simulink model "ipmsm_current_control_CV_FF"  (R2023a)
settings: Solver=FixedStepDiscrete  StartTime=0.0  StopTime=0.8  FixedStep=Ts  RelTol=1e-3  EnableMultiTasking=on
PreLoadFcn:
  | ee_ipmsm_velocity_control_data;
StopFcn:
  | ee_addSimlogTimeStamp(bdroot)
values from neighbouring files (symbols this model uses):
  ActCV = 1    [ipmsm_current_control_data.m]
  down1 = den(1)    [ipmsm_current_control_data.m]
  down2 = den(2)    [ipmsm_current_control_data.m]
  Ki_id = 0.6*Ld/(5*sigma*sigma)    (= 3750)    [ipmsm_current_control_data.m]
  Ki_iq = 0.6*Lq/(5*sigma*sigma)    (= 3750)    [ipmsm_current_control_data.m]
  Kp_id = 0.6*Ld/sigma    (= 1.5)    [ipmsm_current_control_data.m]
  Kp_iq = 0.6*Lq/sigma    (= 1.5)    [ipmsm_current_control_data.m]
  Ld = 0.2e-3    (= 0.0002)    [ipmsm_current_control_data.m]
  Lq = 0.2e-3    (= 0.0002)    [ipmsm_current_control_data.m]
  p = 4    [ipmsm_current_control_data.m]
  Pmax = 1.2*445.3845    (= 534.4614)    [ipmsm_current_control_data.m]
  psim = 0.0064    [ipmsm_current_control_data.m]
  Tmax = 1.2*0.8223    (= 0.98676)    [ipmsm_current_control_data.m]
  Ts = 1e-6    (= 1e-06)    [ipmsm_current_control_data.m]
  Tsi = 5e-5    (= 5e-05)    [ipmsm_current_control_data.m]
  up = num(2)    [ipmsm_current_control_data.m]
  Vnom = 24    [ipmsm_current_control_data.m]
undefined symbols (not defined in the file or in its folder): ee_sli_rtmsupport, gcbh, ID_MAP, IQ_MAP, RPM_VECT, TQ_VECT, VDC_VECT
libraries: nesl_utility x13, fl_lib x10, simulink x10, ee_lib x5, spsMeanLib x4, slpidlib x2, eeDiscretePi x2, eeTransforms x2, eeVelocityController x1, eePwmGeneratorTwoLevel x1, SignalEditorBlockLib x1
(part 2 of 2)

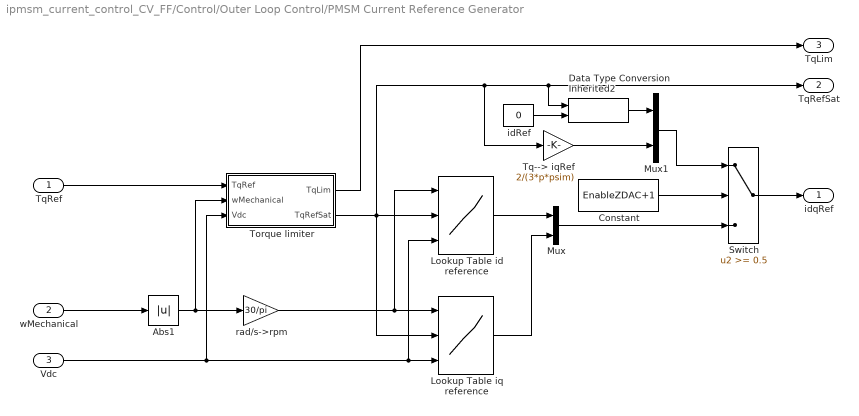
== system ipmsm_current_control_CV_FF/Control/Outer Loop Control/PMSM Current Reference Generator ==
  TqRef : Inport  SampleTime=Ts
  wMechanical : Inport  Port=2  SampleTime=Ts
  Vdc : Inport  Port=3  SampleTime=Ts
  Abs1 : Abs  SaturateOnIntegerOverflow=off
  Constant : Constant  Value=EnableZDAC+1  SampleTime=Ts
  Data Type Conversion Inherited2 : simulink/Signal Attributes/Data Type Conversion Inherited  ConvertRealWorld=Real World Value  DoSatur=off
  Lookup Table id reference : Lookup_n-D  NumberOfTableDimensions=3  BreakpointsForDimension1=rpmVec  BreakpointsForDimension2=TqVec  BreakpointsForDimension3=VdcVec  Table=idMatrix
      settings: InputPortMap=u0,u1,u2
  Lookup Table iq reference : Lookup_n-D  NumberOfTableDimensions=3  BreakpointsForDimension1=rpmVec  BreakpointsForDimension2=TqVec  BreakpointsForDimension3=VdcVec  Table=iqMatrix
      settings: InputPortMap=u0,u1,u2
  Mux : Mux  Inputs=2
  Mux1 : Mux  Inputs=2
  Switch : Switch  Threshold=0.5  SaturateOnIntegerOverflow=off  InputSameDT=off
  Torque limiter : Subsystem
  Tq--> iqRef : Gain  Gain=2/(3*p*psim)
  idRef : Constant  Value=0  SampleTime=Ts
  rad/s->rpm : Gain  Gain=30/pi
  idqRef : Outport  VectorParamsAs1DForOutWhenUnconnected=off
  TqRefSat : Outport  Port=2  VectorParamsAs1DForOutWhenUnconnected=off
  TqLim : Outport  Port=3  VectorParamsAs1DForOutWhenUnconnected=off
  wires:
  idRef/1 -> Data Type Conversion Inherited2/2
  Lookup Table id reference/1 -> Mux/1
  Lookup Table iq reference/1 -> Mux/2
  Torque limiter/2(TqRefSat) -> Lookup Table iq reference/2, Tq--> iqRef/1, TqRefSat/1, Data Type Conversion Inherited2/1, Lookup Table id reference/2
  Torque limiter/1(TqLim) -> TqLim/1
  rad/s->rpm/1 -> Lookup Table id reference/1, Lookup Table iq reference/1
  Abs1/1 -> Torque limiter/2(wMechanical), rad/s->rpm/1
  Mux1/1 -> Switch/1
  Mux/1 -> Switch/3
  Switch/1 -> idqRef/1
  Data Type Conversion Inherited2/1 -> Mux1/1
  Tq--> iqRef/1 -> Mux1/2
  TqRef/1 -> Torque limiter/1(TqRef)
  wMechanical/1 -> Abs1/1
  Vdc/1 -> Lookup Table id reference/3, Lookup Table iq reference/3, Torque limiter/3(Vdc)
  Constant/1 -> Switch/2

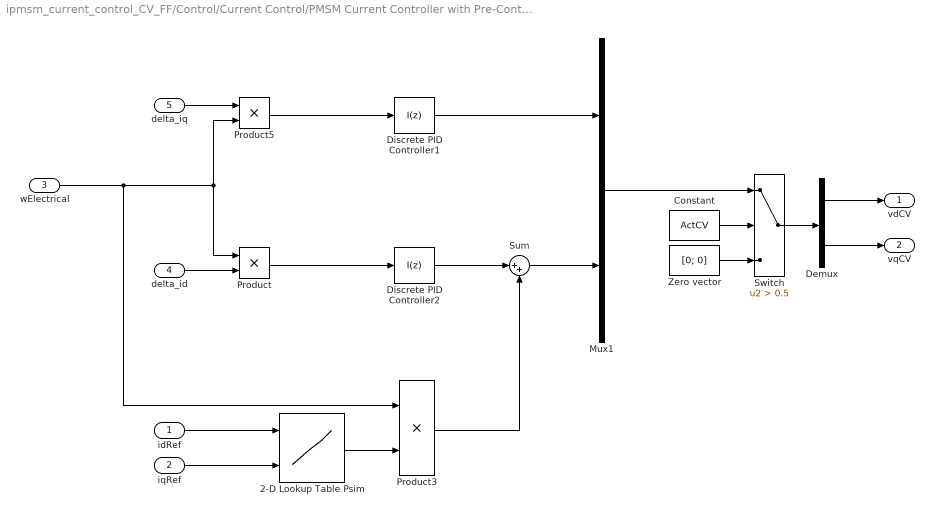
== system ipmsm_current_control_CV_FF/Control/Current Control/PMSM Current Controller with Pre-Control and CV Decoupling/Complex Vector Decoupling ==
  idRef : Inport
  iqRef : Inport  Port=2
  wElectrical : Inport  Port=3
  delta_id : Inport  Port=4
  delta_iq : Inport  Port=5
  2-D Lookup Table Psim : Lookup_n-D  BreakpointsForDimension1=idVect  BreakpointsForDimension2=iqVect  Table=psimMatrix  ExtrapMethod=Clip  InternalRulePriority=Speed  RndMeth=Simplest
      settings: InputPortMap=u0,u1
  Constant : Constant  Value=ActCV  SampleTime=Ts
  Demux : Demux  Outputs=2
  Discrete PID Controller1 : slpidlib/PID Controller  Controller=I  Form=Parallel  TimeDomain=Discrete-time  UseExternalTs=off  SampleTime=Ts  IntegratorMethod=Forward Euler  FilterMethod=Forward Euler  ControllerParametersSource=internal  P=0  I=Kp_iq  UseKiTs=off  D=0  N=100  UseFilter=on  TunerSelectOption=Transfer Function Based (PID Tuner App)  InitialConditionSource=internal  InitialConditionForIntegrator=0  InitialConditionForFilter=0  DifferentiatorICPrevScaledInput=0  ExternalReset=none  TrackingMode=off  Kt=1  LimitOutput=on  SatLimitsSource=internal  UpperSaturationLimit=146.25  LowerSaturationLimit=-146.25  LinearizeAsGain=off  AntiWindupMode=none  Kb=1  LimitIntegrator=off  UpperIntegratorSaturationLimit=inf  LowerIntegratorSaturationLimit=-inf  POutMin=[]  POutMax=[]  IOutMin=[]  IOutMax=[]  DOutMin=[]  DOutMax=[]  NOutMin=[]  NOutMax=[]  SumOutMin=[]  SumOutMax=[]  SaturationOutMin=[]  SaturationOutMax=[]  PParamMin=[]  PParamMax=[]  IParamMin=[]  IParamMax=[]  DParamMin=[]  DParamMax=[]  NParamMin=[]  NParamMax=[]  KbParamMin=[]  KbParamMax=[]  KtParamMin=[]  KtParamMax=[]  KbOutMin=[]  KbOutMax=[]  KtOutMin=[]  KtOutMax=[]  IntegratorOutMin=[]  IntegratorOutMax=[]  FilterOutMin=[]  FilterOutMax=[]  SumI1OutMin=[]  SumI1OutMax=[]  SumI2OutMin=[]  SumI2OutMax=[]  SumI3OutMin=[]  SumI3OutMax=[]  SumI4OutMin=[]  SumI4OutMax=[]  SumDOutMin=[]  SumDOutMax=[]  DifferentiatorOutMin=[]  DifferentiatorOutMax=[]  FilterDiffOutCoefMin=[]  FilterDiffOutCoefMax=[]  ReciprocalOutMin=[]  ReciprocalOutMax=[]  SumDenOutMin=[]  SumDenOutMax=[]  SumNumOutMin=[]  SumNumOutMax=[]  DivideOutMin=[]  DivideOutMax=[]  UdiffTsProdOutMin=[]  UdiffTsProdOutMax=[]  NTsProdOutMin=[]  NTsProdOutMax=[]  UintegralTsProdOutMin=[]  UintegralTsProdOutMax=[]  UngainTsProdOutMin=[]  UngainTsProdOutMax=[]  ClampingZeroOutDataTypeStr=Inherit: Inherit via back propagation  ClampingZeroOutMin=[]  ClampingZeroOutMax=[]  FilterDenConstantOutDataTypeStr=Inherit: Inherit via back propagation  FilterDenConstantOutMin=[]  FilterDenConstantOutMax=[]  PCopyOutDataTypeStr=Inherit: Inherit via back propagation  PCopyOutMin=[]  PCopyOutMax=[]  NCopyOutDataTypeStr=Inherit: Inherit via back propagation  NCopyOutMin=[]  NCopyOutMax=[]  IntegratorContinuousStateAttributes=''  IntegratorStateMustResolveToSignalObject=off  IntegratorRTWStateStorageClass=Auto  FilterContinuousStateAttributes=''  FilterStateMustResolveToSignalObject=off  FilterRTWStateStorageClass=Auto  ParallelPVariant=Disabled  IdealPVariant=Disabled  IVariant=InternalParameters  DVariant=Disabled  IntegratorVariant=Discrete  SatVariant=Enabled  AWVariant=Passthrough  PCopyVariant=Disabled  TRVariant=Disabled  FdbkBlocksVariant=Forward  IdealPFdbkVariant=Disabled  SatFdbkVariant=Disabled  DerivativeFilterVariant=Disabled  NVariant=Disabled  NCopyVariant=Disabled_SignalSpec  FilterICVariant=Disabled  IntegratorICVariant=InternalICs  ExternalResetVariant=Disabled  TRSumVariant=Passthrough  SumFdbkVariant=Disabled  SumVariant=Passthrough_I  TsampFilterVariant=InternalTs  TsampNgainVariant=Passthrough  TsampIntegralVariant=Disabled_SignalSpec  ExternalSaturationOutDataTypeStr=Inherit: Same as second input
  Discrete PID Controller2 : slpidlib/PID Controller  Controller=I  Form=Parallel  TimeDomain=Discrete-time  UseExternalTs=off  SampleTime=Ts  IntegratorMethod=Forward Euler  FilterMethod=Forward Euler  ControllerParametersSource=internal  P=0  I=Kp_id  UseKiTs=off  D=0  N=100  UseFilter=on  TunerSelectOption=Transfer Function Based (PID Tuner App)  InitialConditionSource=internal  InitialConditionForIntegrator=0  InitialConditionForFilter=0  DifferentiatorICPrevScaledInput=0  ExternalReset=none  TrackingMode=off  Kt=1  LimitOutput=on  SatLimitsSource=internal  UpperSaturationLimit=146.25  LowerSaturationLimit=-146.25  LinearizeAsGain=off  AntiWindupMode=none  Kb=1  LimitIntegrator=off  UpperIntegratorSaturationLimit=inf  LowerIntegratorSaturationLimit=-inf  POutMin=[]  POutMax=[]  IOutMin=[]  IOutMax=[]  DOutMin=[]  DOutMax=[]  NOutMin=[]  NOutMax=[]  SumOutMin=[]  SumOutMax=[]  SaturationOutMin=[]  SaturationOutMax=[]  PParamMin=[]  PParamMax=[]  IParamMin=[]  IParamMax=[]  DParamMin=[]  DParamMax=[]  NParamMin=[]  NParamMax=[]  KbParamMin=[]  KbParamMax=[]  KtParamMin=[]  KtParamMax=[]  KbOutMin=[]  KbOutMax=[]  KtOutMin=[]  KtOutMax=[]  IntegratorOutMin=[]  IntegratorOutMax=[]  FilterOutMin=[]  FilterOutMax=[]  SumI1OutMin=[]  SumI1OutMax=[]  SumI2OutMin=[]  SumI2OutMax=[]  SumI3OutMin=[]  SumI3OutMax=[]  SumI4OutMin=[]  SumI4OutMax=[]  SumDOutMin=[]  SumDOutMax=[]  DifferentiatorOutMin=[]  DifferentiatorOutMax=[]  FilterDiffOutCoefMin=[]  FilterDiffOutCoefMax=[]  ReciprocalOutMin=[]  ReciprocalOutMax=[]  SumDenOutMin=[]  SumDenOutMax=[]  SumNumOutMin=[]  SumNumOutMax=[]  DivideOutMin=[]  DivideOutMax=[]  UdiffTsProdOutMin=[]  UdiffTsProdOutMax=[]  NTsProdOutMin=[]  NTsProdOutMax=[]  UintegralTsProdOutMin=[]  UintegralTsProdOutMax=[]  UngainTsProdOutMin=[]  UngainTsProdOutMax=[]  ClampingZeroOutDataTypeStr=Inherit: Inherit via back propagation  ClampingZeroOutMin=[]  ClampingZeroOutMax=[]  FilterDenConstantOutDataTypeStr=Inherit: Inherit via back propagation  FilterDenConstantOutMin=[]  FilterDenConstantOutMax=[]  PCopyOutDataTypeStr=Inherit: Inherit via back propagation  PCopyOutMin=[]  PCopyOutMax=[]  NCopyOutDataTypeStr=Inherit: Inherit via back propagation  NCopyOutMin=[]  NCopyOutMax=[]  IntegratorContinuousStateAttributes=''  IntegratorStateMustResolveToSignalObject=off  IntegratorRTWStateStorageClass=Auto  FilterContinuousStateAttributes=''  FilterStateMustResolveToSignalObject=off  FilterRTWStateStorageClass=Auto  ParallelPVariant=Disabled  IdealPVariant=Disabled  IVariant=InternalParameters  DVariant=Disabled  IntegratorVariant=Discrete  SatVariant=Enabled  AWVariant=Passthrough  PCopyVariant=Disabled  TRVariant=Disabled  FdbkBlocksVariant=Forward  IdealPFdbkVariant=Disabled  SatFdbkVariant=Disabled  DerivativeFilterVariant=Disabled  NVariant=Disabled  NCopyVariant=Disabled_SignalSpec  FilterICVariant=Disabled  IntegratorICVariant=InternalICs  ExternalResetVariant=Disabled  TRSumVariant=Passthrough  SumFdbkVariant=Disabled  SumVariant=Passthrough_I  TsampFilterVariant=InternalTs  TsampNgainVariant=Passthrough  TsampIntegralVariant=Disabled_SignalSpec  ExternalSaturationOutDataTypeStr=Inherit: Same as second input
  Mux1 : Mux  Inputs=2
  Product : Product
  Product3 : Product
  Product5 : Product
  Sum : Sum  Inputs=|++
  Switch : Switch  Criteria=u2 > Threshold  Threshold=0.5  SaturateOnIntegerOverflow=off  InputSameDT=off  OutDataTypeStr=Inherit: Same as first input
  Zero vector : Constant  Value=[0; 0]  SampleTime=Ts
  vdCV : Outport  VectorParamsAs1DForOutWhenUnconnected=off
  vqCV : Outport  Port=2  VectorParamsAs1DForOutWhenUnconnected=off
  wires:
  Switch/1 -> Demux/1
  Demux/2 -> vqCV/1
  Constant/1 -> Switch/2
  Mux1/1 -> Switch/1
  Demux/1 -> vdCV/1
  Zero vector/1 -> Switch/3
  Product/1 -> Discrete PID Controller2/1
  Product5/1 -> Discrete PID Controller1/1
  Discrete PID Controller2/1 -> Sum/1
  idRef/1 -> 2-D Lookup Table Psim/1
  iqRef/1 -> 2-D Lookup Table Psim/2
  delta_iq/1 -> Product5/1
  delta_id/1 -> Product/2
  wElectrical/1 -> Product3/1, Product/1, Product5/2
  2-D Lookup Table Psim/1 -> Product3/2
  Product3/1 -> Sum/2
  Sum/1 -> Mux1/2
  Discrete PID Controller1/1 -> Mux1/1

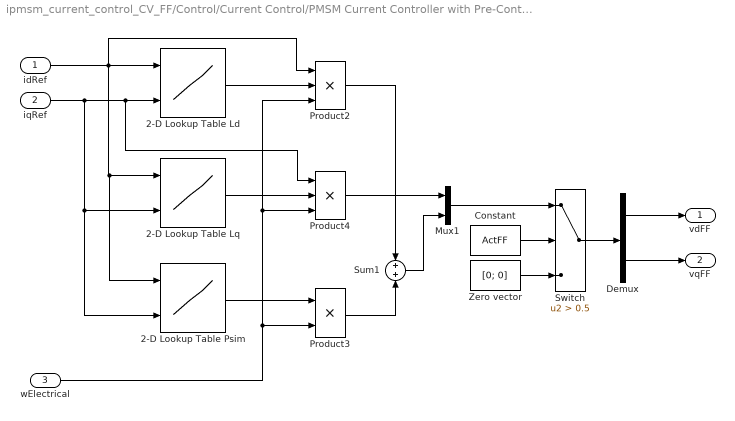
== system ipmsm_current_control_CV_FF/Control/Current Control/PMSM Current Controller with Pre-Control and CV Decoupling/Feedforward pre-control ==
  idRef : Inport
  iqRef : Inport  Port=2
  wElectrical : Inport  Port=3
  2-D Lookup Table Ld : Lookup_n-D  BreakpointsForDimension1=idVect  BreakpointsForDimension2=iqVect  Table=LdMatrix  ExtrapMethod=Clip  UseLastTableValue=on  InternalRulePriority=Speed  RndMeth=Simplest
      settings: InputPortMap=u0,u1
  2-D Lookup Table Lq : Lookup_n-D  BreakpointsForDimension1=idVect  BreakpointsForDimension2=iqVect  Table=LqMatrix  ExtrapMethod=Clip  InternalRulePriority=Speed  RndMeth=Simplest
      settings: InputPortMap=u0,u1
  2-D Lookup Table Psim : Lookup_n-D  BreakpointsForDimension1=idVect  BreakpointsForDimension2=iqVect  Table=psimMatrix  ExtrapMethod=Clip  InternalRulePriority=Speed  RndMeth=Simplest
      settings: InputPortMap=u0,u1
  Constant : Constant  Value=ActFF  SampleTime=Ts
  Demux : Demux  Outputs=2
  Mux1 : Mux  Inputs=2
  Product2 : Product  Inputs=3
  Product3 : Product
  Product4 : Product  Inputs=3
  Sum1 : Sum
  Switch : Switch  Criteria=u2 > Threshold  Threshold=0.5  SaturateOnIntegerOverflow=off  InputSameDT=off  OutDataTypeStr=Inherit: Same as first input
  Zero vector : Constant  Value=[0; 0]  SampleTime=Ts
  vdFF : Outport  VectorParamsAs1DForOutWhenUnconnected=off
  vqFF : Outport  Port=2  VectorParamsAs1DForOutWhenUnconnected=off
  wires:
  Product2/1 -> Sum1/1
  wElectrical/1 -> Product2/3, Product4/3, Product3/2
  Mux1/1 -> Switch/1
  Product4/1 -> Mux1/1
  idRef/1 -> 2-D Lookup Table Ld/1, 2-D Lookup Table Lq/1, 2-D Lookup Table Psim/1, Product2/1
  iqRef/1 -> 2-D Lookup Table Psim/2, 2-D Lookup Table Lq/2, 2-D Lookup Table Ld/2, Product4/1
  2-D Lookup Table Ld/1 -> Product2/2
  Sum1/1 -> Mux1/2
  Zero vector/1 -> Switch/3
  2-D Lookup Table Psim/1 -> Product3/1
  Demux/2 -> vqFF/1
  Demux/1 -> vdFF/1
  Switch/1 -> Demux/1
  Constant/1 -> Switch/2
  2-D Lookup Table Lq/1 -> Product4/2
  Product3/1 -> Sum1/2

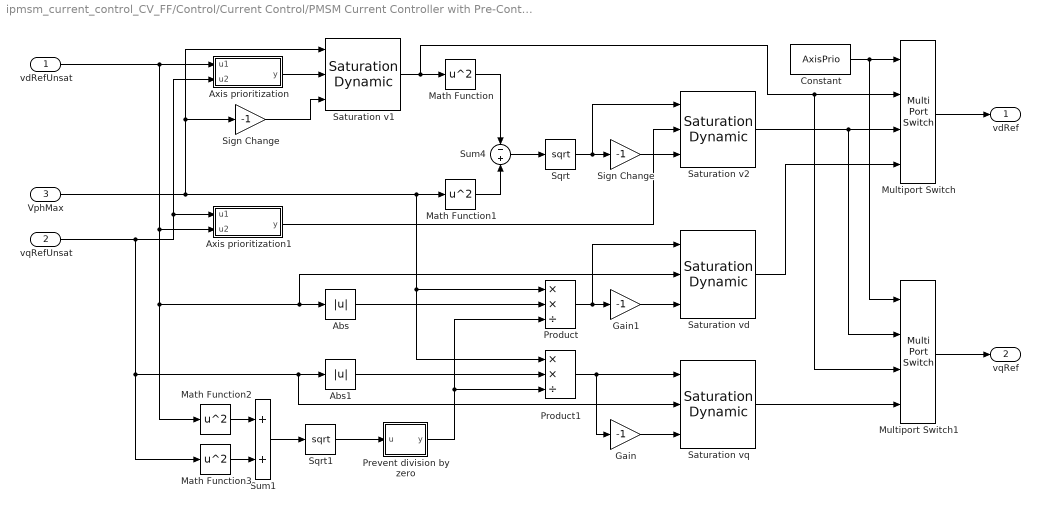
== system ipmsm_current_control_CV_FF/Control/Current Control/PMSM Current Controller with Pre-Control and CV Decoupling/d-q Voltage Limiter ==
  vdRefUnsat : Inport  SampleTime=Ts
  vqRefUnsat : Inport  Port=2  SampleTime=Ts
  VphMax : Inport  Port=3  SampleTime=Ts
  Abs : Abs  SaturateOnIntegerOverflow=off
  Abs1 : Abs  SaturateOnIntegerOverflow=off
  Axis prioritization : Subsystem
  Axis prioritization1 : Subsystem
  Constant : Constant  Value=AxisPrio  SampleTime=Ts
  Gain : Gain  Gain=-1
  Gain1 : Gain  Gain=-1
  Math Function{,1..3} (4 alike) : Math  Operator=square  SignedPower=on
  Multiport Switch : MultiPortSwitch  DiagnosticForDefault=Warning  SaturateOnIntegerOverflow=off  InputSameDT=off
  Multiport Switch1 : MultiPortSwitch  DiagnosticForDefault=Warning  SaturateOnIntegerOverflow=off  InputSameDT=off
  Prevent division by zero : Subsystem
  Product : Product  Inputs=**/
  Product1 : Product  Inputs=**/
  Saturation v1 : simulink/Discontinuities/Saturation Dynamic  OutMin=[]  OutMax=[]  OutDataTypeStr=Inherit: Same as second input  OutDataType=fixdt(1, 16)  OutScaling=2^-10  DoSatur=off
  Saturation v2 : simulink/Discontinuities/Saturation Dynamic  OutMin=[]  OutMax=[]  OutDataTypeStr=Inherit: Same as second input  OutDataType=fixdt(1, 16)  OutScaling=2^-10  DoSatur=off
  Saturation vd : simulink/Discontinuities/Saturation Dynamic  OutMin=[]  OutMax=[]  OutDataTypeStr=Inherit: Same as second input  OutDataType=fixdt(1, 16)  OutScaling=2^-10  DoSatur=off
  Saturation vq : simulink/Discontinuities/Saturation Dynamic  OutMin=[]  OutMax=[]  OutDataTypeStr=Inherit: Same as second input  OutDataType=fixdt(1, 16)  OutScaling=2^-10  DoSatur=off
  Sign Change : Gain  Gain=-1
  "Sign Change " : Gain  Gain=-1
  Sqrt : Sqrt
  Sqrt1 : Sqrt
  Sum1 : Sum
  Sum4 : Sum  Inputs=-+
  vdRef : Outport  VectorParamsAs1DForOutWhenUnconnected=off
  vqRef : Outport  Port=2  VectorParamsAs1DForOutWhenUnconnected=off
  wires:
  "Sign Change "/1 -> Saturation v2/3
  Sqrt/1 -> "Sign Change "/1, Saturation v2/1
  Math Function/1 -> Sum4/1
  Sum4/1 -> Sqrt/1
  Math Function1/1 -> Sum4/2
  Sign Change/1 -> Saturation v1/3
  Saturation v1/1 -> Multiport Switch1/3, Multiport Switch/2, Math Function/1
  Axis prioritization1/1(y) -> Saturation v2/2
  Axis prioritization/1(y) -> Saturation v1/2
  vqRefUnsat/1 -> Saturation vq/2, Abs1/1, Math Function3/1, Axis prioritization1/1(u1), Axis prioritization/2(u2)
  Sum1/1 -> Sqrt1/1
  VphMax/1 -> Math Function1/1, Product1/1, Product/1, Saturation v1/1, Sign Change/1
  vdRefUnsat/1 -> Axis prioritization/1(u1), Math Function2/1, Saturation vd/2, Abs/1, Axis prioritization1/2(u2)
  Math Function2/1 -> Sum1/1
  Math Function3/1 -> Sum1/2
  Sqrt1/1 -> Prevent division by zero/1(u)
  Constant/1 -> Multiport Switch1/1, Multiport Switch/1
  Saturation v2/1 -> Multiport Switch/3, Multiport Switch1/2
  Multiport Switch/1 -> vdRef/1
  Multiport Switch1/1 -> vqRef/1
  Prevent division by zero/1(y) -> Product/3, Product1/3
  Abs/1 -> Product/2
  Abs1/1 -> Product1/2
  Product/1 -> Saturation vd/1, Gain1/1
  Product1/1 -> Saturation vq/1, Gain/1
  Saturation vq/1 -> Multiport Switch1/4
  Saturation vd/1 -> Multiport Switch/4
  Gain/1 -> Saturation vq/3
  Gain1/1 -> Saturation vd/3

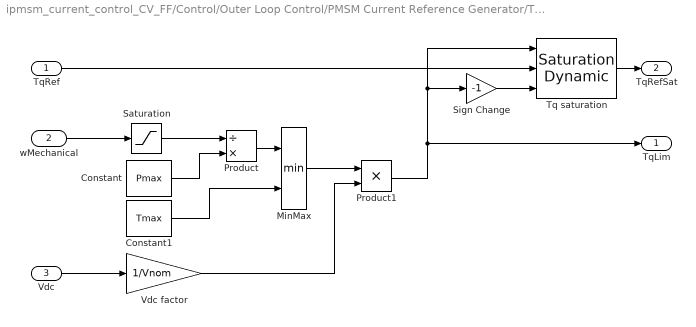
== system ipmsm_current_control_CV_FF/Control/Outer Loop Control/PMSM Current Reference Generator/Torque limiter ==
  TqRef : Inport
  wMechanical : Inport  Port=2
  Vdc : Inport  Port=3
  Constant : Constant  Value=Pmax  SampleTime=Ts
  Constant1 : Constant  Value=Tmax  SampleTime=Ts
  MinMax : MinMax  Inputs=2  OutDataTypeStr=Inherit: Same as first input
  Product : Product  Inputs=/*  OutDataTypeStr=Inherit: Same as first input
  Product1 : Product
  Saturation : Saturate  UpperLimit=inf  LowerLimit=Pmax/Tmax
  Sign Change : Gain  Gain=-1
  Tq saturation : simulink/Discontinuities/Saturation Dynamic  OutMin=[]  OutMax=[]  OutDataTypeStr=Inherit: Same as second input  OutDataType=fixdt(1, 16)  OutScaling=2^-10  DoSatur=off
  Vdc factor : Gain  Gain=1/Vnom
  TqLim : Outport  VectorParamsAs1DForOutWhenUnconnected=off
  TqRefSat : Outport  Port=2  VectorParamsAs1DForOutWhenUnconnected=off
  wires:
  Constant/1 -> Product/2
  Saturation/1 -> Product/1
  Tq saturation/1 -> TqRefSat/1
  Product1/1 -> Tq saturation/1, Sign Change/1, TqLim/1
  TqRef/1 -> Tq saturation/2
  Vdc/1 -> Vdc factor/1
  Constant1/1 -> MinMax/2
  wMechanical/1 -> Saturation/1
  Product/1 -> MinMax/1
  Sign Change/1 -> Tq saturation/3
  MinMax/1 -> Product1/1
  Vdc factor/1 -> Product1/2

== system ipmsm_current_control_CV_FF/Control/Current Control/PMSM Current Controller with Pre-Control and CV Decoupling/d-q Voltage Limiter/Axis prioritization ==
  u1 : Inport
  u2 : Inport  Port=2
  Compare To Constant : simulink/Logic and Bit Operations/Compare To Constant  relop===  const=1  OutDataTypeStr=boolean
  Constant : Constant  Value=AxisPrio  SampleTime=Ts
  Switch : Switch  Criteria=u2 ~= 0  Threshold=1  SaturateOnIntegerOverflow=off  InputSameDT=off
  y : Outport  VectorParamsAs1DForOutWhenUnconnected=off
  wires:
  u1/1 -> Switch/1
  u2/1 -> Switch/3
  Switch/1 -> y/1
  Constant/1 -> Compare To Constant/1
  Compare To Constant/1 -> Switch/2

== system ipmsm_current_control_CV_FF/Control/Current Control/PMSM Current Controller with Pre-Control and CV Decoupling/d-q Voltage Limiter/Axis prioritization1 ==
  u1 : Inport
  u2 : Inport  Port=2
  Compare To Constant : simulink/Logic and Bit Operations/Compare To Constant  relop===  const=1  OutDataTypeStr=boolean
  Constant : Constant  Value=AxisPrio  SampleTime=Ts
  Switch : Switch  Criteria=u2 ~= 0  Threshold=1  SaturateOnIntegerOverflow=off  InputSameDT=off
  y : Outport  VectorParamsAs1DForOutWhenUnconnected=off
  wires:
  u1/1 -> Switch/1
  u2/1 -> Switch/3
  Switch/1 -> y/1
  Compare To Constant/1 -> Switch/2
  Constant/1 -> Compare To Constant/1

== system ipmsm_current_control_CV_FF/Control/Current Control/PMSM Current Controller with Pre-Control and CV Decoupling/d-q Voltage Limiter/Prevent division by zero ==
  u : Inport
  Constant1 : Constant  Value=0.001
  Data Type Conversion Inherited : simulink/Signal Attributes/Data Type Conversion Inherited  ConvertRealWorld=Real World Value  DoSatur=off
  Switch : Switch  Criteria=u2 > Threshold  Threshold=0.001  SaturateOnIntegerOverflow=off  InputSameDT=off
  y : Outport  VectorParamsAs1DForOutWhenUnconnected=off
  wires:
  u/1 -> Data Type Conversion Inherited/1, Switch/1, Switch/2
  Switch/1 -> y/1
  Data Type Conversion Inherited/1 -> Switch/3
  Constant1/1 -> Data Type Conversion Inherited/2
